simulink model "Mixed_Radix_IFFT_Ex1"  (R2022a)
settings: Solver=VariableStepAuto  StartTime=0.0  StopTime=1  RelTol=1e-3
undefined symbols (not defined in the file): None, Radix, S, vsva2197, xcvc1902
libraries: dspxfrm3 x2, dspsrcs4 x1, aieDSP x1, vmcUtilities x1
settings Model: Creator=sdegala  LastModifiedBy=sdegala

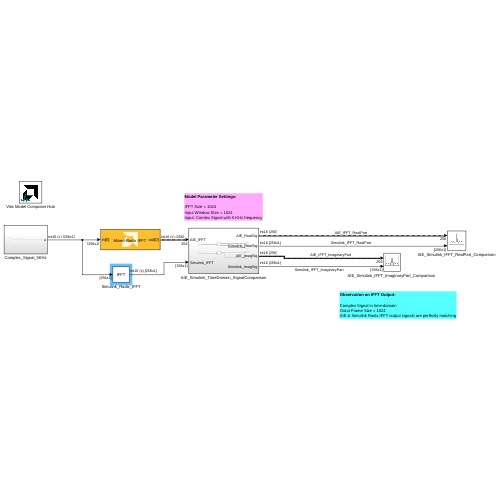
[thumbnail: Simulink's stored preview of the top-level diagram]
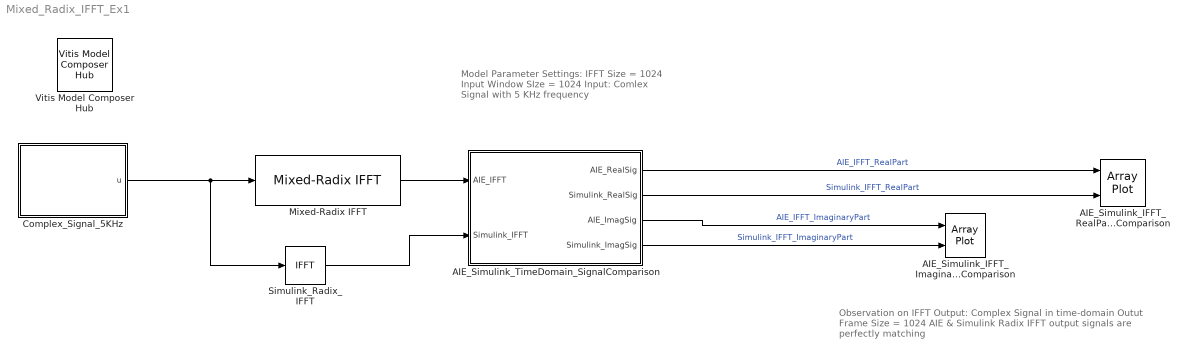
== system Mixed_Radix_IFFT_Ex1 ==
  note: Model Parameter Settings:
      |
      | IFFT Size = 1024
      | Input Window SIze = 1024
      | Input: Comlex Signal with 5 KHz frequency
  note: Observation on IFFT Output:
      |
      | Complex Signal in time-domain
      | Outut Frame Size = 1024
      | AIE & Simulink Radix IFFT output signals are perfectly matching
  "AIE_Simulink_IFFT_ImaginaryPart_Comparison " : ArrayPlot  NumInputPorts=2  WindowPosition=[134.000000,82.000000,1061.000000,557.000000,]  ScopeFrameLocation=window  PlotType=Line  AxesScaling=Manual  YLimits=[-1000,1000]  ShowLegend=on
  AIE_Simulink_IFFT_RealPart_Comparison : ArrayPlot  NumInputPorts=2  WindowPosition=[1.000000,37.000000,1280.000000,655.000000,]  ScopeFrameLocation=window  PlotType=Line  YLimits=[-1280,1280]  ShowLegend=on
  AIE_Simulink_TimeDomain_SignalComparison : Subsystem
  Complex_Signal_5KHz : Subsystem
  Mixed-Radix IFFT : aieDSP/Mixed-Radix IFFT  data_type=cint16  twiddle_type=cint16  point_size=1024  input_window_size=1024  shift_val=0  rnd_mode=Round symmetrical to infinity  sat_mode=0-None  casc_length=1  blockJsonConstraints=[]  blockJsonConstraintsInternal=[]  spec=vmc_mixed_radix_ifft.json  SerializedMaskParamNames=[]  SerializedMaskParamValues=[]  SerializedMaskParamVisibilities=[]  block_type=Mixed-Radix IFFT  SerializedMaskParamDataypes=typename|typename|uint|uint|uint|uint|uint|uint  SerializedMaskParamEnumStrArr=0|0|0|0|0|Floor,Ceiling,Round to positive infinity,Round to negative infinity,Round symmetrical to infinity,Round symmetrical to zero,Round convergent to even,Round convergent to odd|0-None,1-Asymmetric,3-Symmetric|0  SerializedMaskParamEnumValArr=0|0|0|0|0|0,1,2,3,4,5,6,7|0,1,3|0  SerializedMaskParamVectorArr=0|0|0|0|0|0|0|0
  Simulink_Radix_IFFT : dspxfrm3/IFFT  FFTImplementation=Radix-2  CompMethod=Table lookup  TableOpt=NEW  TableOptActive=Speed  BitRevOrder=off  cs_in=off  Normalize=off  InheritFFTLength=on  FFTLength=64  WrapInput=on  mode=Complex  outSamplingMode=Sample based  roundingMode=Floor  overflowMode=off  firstCoeffDataTypeStr=Inherit: Same word length as input  firstCoeffLastDataTypeStr=Inherit: Same word length as input  prodOutputMode=Binary point scaling  prodOutputWordLength=24  prodOutputFracLength=0  prodOutputDataTypeStr=fixdt(1,24,0)  prodOutputLastDataTypeStr=fixdt(1,24,0)  outputMode=Binary point scaling  outputWordLength=16  outputFracLength=0  outputDataTypeStr=fixdt(1,16,0)  outputMin=[]  outputMax=[]  outputLastDataTypeStr=fixdt(1,16,0)
  Vitis Model Composer Hub : vmcUtilities/Vitis Model Composer Hub  Tag=genX  CodeGeneration=off  TargetDirectory=./code  ExportType=AI Engines  IpVendor=xilinx.com  IpLibrary=hls  IpVersion=1.0  IpHWLanguage=Verilog  AieCompilerOptions={}  AieSimulatorOptions={}  CreateTestbench=off  TestbenchStackSize=10  RunRtlSim=off  RunCSim=off  RunAieSim=off  AieSimTimeout=50000  RunAieSimProfiling=off  LaunchVitisAnalyzer=off  PlotOutput=off  RunX86Sim=off  X86SimTimeout=10  GenHwImage=off  GenLibadfXo=off  PlatformType=Not Specified  HwSystemType=Baremetal  HwValidationTarget=hw  ProjDevice=xcvc1902-vsva2197-1LP-e-S  ProjDevicePart=xcvc1902-vsva2197-1LP-e-S  AIEType=AIE  SamplePeriod=-1  ClockFrequency=200  DataPathParallelism=1  xilinxfamily=versalaicore  part=xcvc1902  speed=-1LP-e-S  package=vsva2197  directory=./netlist  testbench=off  incr_netlist=off  synthesis_tool=Vivado  clock_wrapper=Clock Enables  dbl_ovrd=According to Block Masks  dcm_input_clock_period=10  sysclk_period=10  simulink_period=1  eval_field=0  LogFileName=''  NThreads=4
  wires:
  Complex_Signal_5KHz/1(u) -> Simulink_Radix_IFFT/1, Mixed-Radix IFFT/1
  Mixed-Radix IFFT/1 -> AIE_Simulink_TimeDomain_SignalComparison/1(AIE_IFFT)
  Simulink_Radix_IFFT/1 -> AIE_Simulink_TimeDomain_SignalComparison/2(Simulink_IFFT)
  AIE_Simulink_TimeDomain_SignalComparison/1(AIE_RealSig) -> AIE_Simulink_IFFT_RealPart_Comparison/1  "AIE_IFFT_RealPart"
  AIE_Simulink_TimeDomain_SignalComparison/2(Simulink_RealSig) -> AIE_Simulink_IFFT_RealPart_Comparison/2  "Simulink_IFFT_RealPart"
  AIE_Simulink_TimeDomain_SignalComparison/3(AIE_ImagSig) -> "AIE_Simulink_IFFT_ImaginaryPart_Comparison "/1  "AIE_IFFT_ImaginaryPart"
  AIE_Simulink_TimeDomain_SignalComparison/4(Simulink_ImagSig) -> "AIE_Simulink_IFFT_ImaginaryPart_Comparison "/2  "Simulink_IFFT_ImaginaryPart"

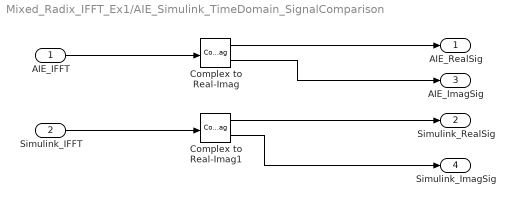
== system Mixed_Radix_IFFT_Ex1/AIE_Simulink_TimeDomain_SignalComparison ==
  AIE_IFFT : Inport
  Simulink_IFFT : Inport  Port=2
  Complex to Real-Imag : ComplexToRealImag
  Complex to Real-Imag1 : ComplexToRealImag
  AIE_RealSig : Outport
  Simulink_RealSig : Outport  Port=2
  AIE_ImagSig : Outport  Port=3
  Simulink_ImagSig : Outport  Port=4
  wires:
  AIE_IFFT/1 -> Complex to Real-Imag/1
  Complex to Real-Imag/1 -> AIE_RealSig/1
  Complex to Real-Imag1/1 -> Simulink_RealSig/1
  Complex to Real-Imag1/2 -> Simulink_ImagSig/1
  Complex to Real-Imag/2 -> AIE_ImagSig/1
  Simulink_IFFT/1 -> Complex to Real-Imag1/1

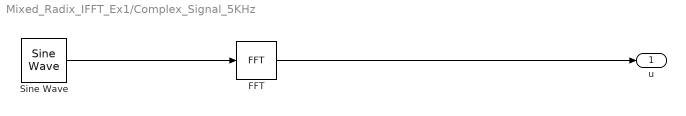
== system Mixed_Radix_IFFT_Ex1/Complex_Signal_5KHz ==
  FFT : dspxfrm3/FFT  FFTImplementation=Radix-2  CompMethod=Table lookup  TableOpt=NEW  TableOptActive=Speed  BitRevOrder=off  Normalize=off  InheritFFTLength=on  FFTLength=64  WrapInput=on  roundingMode=Floor  overflowMode=off  firstCoeffDataTypeStr=Inherit: Same word length as input  firstCoeffLastDataTypeStr=Inherit: Same word length as input  outputMode=Binary point scaling  outputWordLength=16  outputFracLength=0  outputDataTypeStr=fixdt(1,16,0)  outputMin=[]  outputMax=[]  outputLastDataTypeStr=fixdt(1,16,0)
  Sine Wave : dspsrcs4/Sine Wave  Amplitude=1  Frequency=5e3  Phase=0  SampleMode=Discrete  OutComplex=Complex  CompMethod=Table lookup  TableSize=Speed  SampleTime=1/20e3  SamplesPerFrame=1024  ResetState=Restart at time zero  OutputFrames=off  dataType=Fixed-point  wordLen=16  udDataType=sfix(16)  fracBitsMode=User-defined  numFracBits=14  OutDataTypeStr=fixdt(1,16,14)  LastOutDataTypeStr=fixdt(1,16,14)
  u : Outport
  wires:
  Sine Wave/1 -> FFT/1
  FFT/1 -> u/1
